simulink model "Simula"  (R2018a)
settings: Solver=FixedStepDiscrete  StartTime=0.0  StopTime=(length(SG))/FS  RelTol=1e-3
values from neighbouring files (symbols this model uses):
  FS = 1    [MAIN.m]
  SG = [G]    [MAIN.m]
  ST = [T]    [MAIN.m]
libraries: powerlib_meascontrol x7, dspindex x2
settings Model: Creator=USUARIO  LastModifiedBy=USUARIO
settings DataIOCC: SaveOutput=off  SignalLogging=off  DSMLogging=off  SaveTime=off

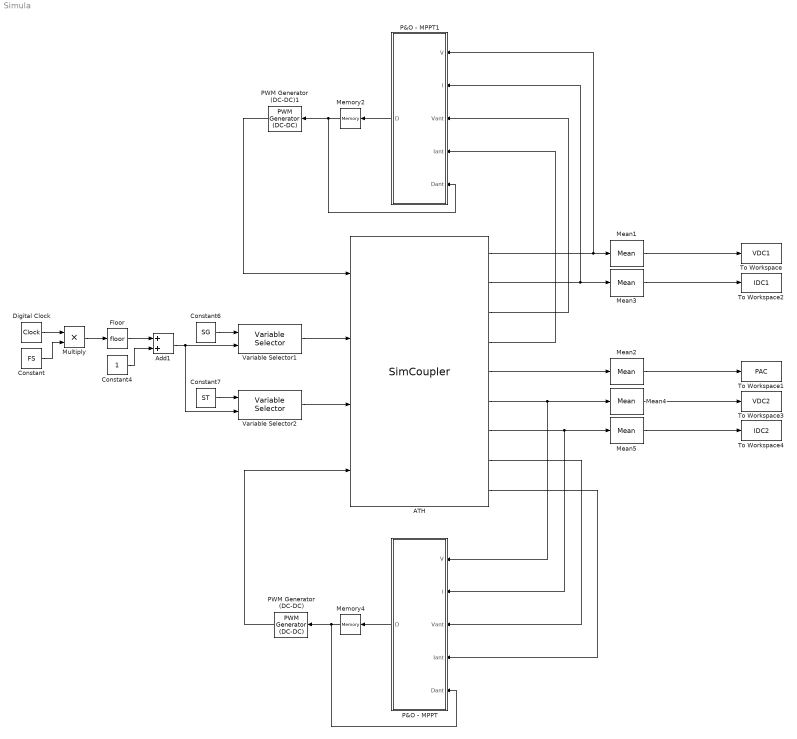
== system Simula ==
  ATH : S-Function  FunctionName=SimCoupler  Parameters=PATH  SFunctionDeploymentMode=off  EnableBusSupport=off
      mask init:
      | x1=1;y1=1;x2=1;y2=1;
      settings: OpenFcn=PsimDialog('PSimFileEdt','Value','Parameters');  CloseFcn=close(gcf);
      mask Display: plot(-60,-60,60,60,x1,y1,x2,y2)
  Add1 : Sum
  Constant : Constant  Value=FS
  Constant4 : Constant
  Constant6 : Constant  Value=SG
  Constant7 : Constant  Value=ST
  Digital Clock : DigitalClock  SampleTime=5e-5
  Floor : Rounding
  Mean{1..5} (5 alike) : powerlib_meascontrol/Measurements/Mean  Freq=FS*4  Vinit=0  Ts=0.05
  Memory2 : Memory  InitialCondition=0.5  LinearizeMemory=on
  Memory4 : Memory  InitialCondition=0.5  LinearizeMemory=on
  Multiply : Product
  P&O - MPPT : MATLAB Function  TreatAsAtomicUnit=on
  P&O - MPPT1 : MATLAB Function  TreatAsAtomicUnit=on
  PWM Generator (DC-DC) : powerlib_meascontrol/Pulse & Signal Generators/PWM Generator (DC-DC)  Fsw=1000  Ts=0
  PWM Generator (DC-DC)1 : powerlib_meascontrol/Pulse & Signal Generators/PWM Generator (DC-DC)  Fsw=1000  Ts=0
  To Workspace : ToWorkspace  VariableName=VDC1  SampleTime=1/FS
  To Workspace1 : ToWorkspace  VariableName=PAC  SampleTime=1/FS
  To Workspace2 : ToWorkspace  VariableName=IDC1  SampleTime=1/FS
  To Workspace3 : ToWorkspace  VariableName=VDC2  SampleTime=1/FS
  To Workspace4 : ToWorkspace  VariableName=IDC2  SampleTime=1/FS
  Variable Selector1 : dspindex/Variable Selector  NumInputs=1  rowsOrCols=Rows  IdxMode=Variable  Elements=[1 3]  ZerOneIdxMode=One-based  errmode=Clip Index  FillMode=on  FillValues=0
  Variable Selector2 : dspindex/Variable Selector  NumInputs=1  rowsOrCols=Rows  IdxMode=Variable  Elements=[1 3]  ZerOneIdxMode=One-based  errmode=Clip Index  FillMode=on  FillValues=0
  wires:
  Constant4/1 -> Add1/2
  Floor/1 -> Add1/1
  Constant6/1 -> Variable Selector1/1
  Add1/1 -> Variable Selector1/2, Variable Selector2/2
  Constant7/1 -> Variable Selector2/1
  Multiply/1 -> Floor/1
  P&O - MPPT/1(D) -> Memory4/1
  Variable Selector2/1 -> ATH/3
  Variable Selector1/1 -> ATH/2
  P&O - MPPT1/1(D) -> Memory2/1
  Memory2/1 -> PWM Generator (DC-DC)1/1, P&O - MPPT1/5(Dant)
  ATH/1 -> P&O - MPPT1/1(V), Mean1/1
  ATH/2 -> P&O - MPPT1/2(I), Mean3/1
  ATH/3 -> P&O - MPPT1/3(Vant)
  ATH/4 -> P&O - MPPT1/4(Iant)
  ATH/5 -> Mean2/1
  PWM Generator (DC-DC)1/1 -> ATH/1
  Memory4/1 -> PWM Generator (DC-DC)/1, P&O - MPPT/5(Dant)
  PWM Generator (DC-DC)/1 -> ATH/4
  ATH/6 -> P&O - MPPT/1(V), Mean4/1
  ATH/7 -> Mean5/1, P&O - MPPT/2(I)
  ATH/9 -> P&O - MPPT/4(Iant)
  ATH/8 -> P&O - MPPT/3(Vant)
  Mean3/1 -> To Workspace2/1
  Mean2/1 -> To Workspace1/1
  Mean4/1 -> To Workspace3/1
  Mean5/1 -> To Workspace4/1
  Digital Clock/1 -> Multiply/1
  Constant/1 -> Multiply/2
  Mean1/1 -> To Workspace/1

== matlab function Simula/P&O - MPPT1 ==
  data: V input; D output; I input; Vant input; Iant input; Dant input
function D = fcn(V, I, Vant, Iant, Dant)

P=V*I;
Pant=Vant*Iant;
m=-0.00001;

if P>Pant
    if V>Vant
        D=Dant+m;
    else
        D=Dant-m;
    end
elseif P<Pant
    if V>Vant
        D=Dant-m;
    else
        D=Dant+m;
    end
else
    D=Dant;
end

if D>1
    D=1;
end
if D<0
    D=0;
end

== matlab function Simula/P&O - MPPT ==
  data: V input; D output; I input; Vant input; Iant input; Dant input
function D = fcn(V, I, Vant, Iant, Dant)

P=V*I;
Pant=Vant*Iant;
m=-0.00001;

if P>Pant
    if V>Vant
        D=Dant+m;
    else
        D=Dant-m;
    end
elseif P<Pant
    if V>Vant
        D=Dant-m;
    else
        D=Dant+m;
    end
else
    D=Dant;
end

if D>1
    D=1;
end
if D<0
    D=0;
end
